simulink model "PassVeh3DOF"  (R2020a)
settings: Solver=ode4  StartTime=0.0  StopTime=10  FixedStep=.001  RelTol=3e-3
model workspace (MAT data in the model file):
  A_mu = 10
  B_reff = 8.386
  CONVERTER_DATA = [0 0.1 0.2 0.3 0.4 0.5 0.6 0.7 0.8 0.81 0.82 0.83 ... (63 elements, 21x3)]
  Cps = 2
  Cz = 7766.25
  DOWN_TABLE = [0 0 0 0 0 0 5 5 7.5 7.5 15 15 ... (30 elements, 6x5)]
  DOWN_TH_BP = [0 5 40 50 90 100]
  D_reff = 0.25826
  EMAP = [-40 215 245 264 264 267 267 267 267 267 -44 117 ... (110 elements, 10x11)]
  F0z = [6086.4 4324.8]
  F_reff = 0.07394
  F_zmax = 10000
  F_zmin = 100
  F_zo = 4000
  Kz = 48000
  MF : object (value not decoded)
  NCyl = 6
  NE_VEC = [800 1200 1600 2000 2400 2800 3200 3600 4000 4400 4800]
  Pstd = 101325
  Rair = 287
  SUS : object (value not decoded)
  TH_VEC = [0; 20; 30; 40; 50; 60; 70; 80; 90; 100]
  TWAITdn = 1.25
  TWAITup = 0.1
  Tin = [1 2 3 4 5 6 7 8 9 10 2 2 ... (20 elements, 10x2)]
  Tstd = 293.15
  UP_TABLE = [7.5 7.5 15 25 40 40 25 25 35 45 70 80 ... (30 elements, 6x5)]
  UP_TH_BP = [0 25 35 50 90 100]
  VEH : object (value not decoded)
  V_o = 16.7
  V_xlow = 1
  Vd = 0.00346
  WH : object (value not decoded)
  a = 1.4
  alpha_max = 1.5
  alpha_min = -1.5
  b = 1.8
  c_zo = 209651
  epsilon = 0.1
  f_air = [0 0 0 0 0 0 0 0 0 0 0 0 ... (256 elements, 16x16)]
  f_co = [0 0 0 0 0 0 0 0 0 0 0 0 ... (256 elements, 16x16)]
  f_co2 = [0 0 0 0 0 0 0 0 0 0 0 0 ... (256 elements, 16x16)]
  f_eff = [352.135682859 352.135682859 320.724378192 303.655312657 295.930136708 291.240087194 291.240271258 291.240312459 291.240275452 291.240198499 291.240100781 291.240018769 ... (256 elements, 16x16)]
  f_fuel = [0 0 0 0 0 0 0 0 0 0 0 0 ... (256 elements, 16x16)]
  f_hc = [0 0 0 0 0 0 0 0 0 0 0 0 ... (256 elements, 16x16)]
  f_nox = [0 0 0 0 0 0 0 0 0 0 0 0 ... (256 elements, 16x16)]
  f_pm = [0 0 0 0 0 0 0 0 0 0 0 0 ... (256 elements, 16x16)]
  f_susp_axl_bp = [1 2]
  f_susp_dz_bp = [-4 -0.14 -0.13 -0.12 -0.11 -0.1 -0.09 -0.08 -0.07 -0.06 -0.05 -0.04 ... (31 elements, 1x31)]
  f_susp_dzdot_bp = [-4 -0.14 -0.13 -0.12 -0.11 -0.1 -0.09 -0.08 -0.07 -0.06 -0.05 -0.04 ... (31 elements, 1x31)]
  f_susp_fmz = [-213379.591456 -28099.591456 -27619.591456 -27139.591456 -26659.591456 -26179.591456 -25699.591456 -25219.591456 -24739.591456 -24259.591456 -23779.591456 -23299.591456 ... (468968 elements, 31x31x61x2x4)]
  f_susp_geom = [-0.832564012244 0.043269987756 0.045538987756 0.047807987756 0.050076987756 0.052345987756 0.054614987756 0.056883987756 0.059152987756 0.061421987756 0.063690987756 0.065959987756 ... (11346 elements, 31x61x2x3)]
  f_susp_strgdelta_bp = [-0.523598775598 -0.506145483078 -0.488692190558 -0.471238898038 -0.453785605519 -0.436332312999 -0.418879020479 -0.401425727959 -0.383972435439 -0.366519142919 -0.349065850399 -0.331612557879 ... (61 elements, 1x61)]
  f_tbrake = [0 76.8593923996 105.140482948 131.533638111 157.926793274 176.658631717 176.65727296 176.656856686 176.656879077 176.657093756 176.657404516 176.65772406 ... (256 elements, 16x16)]
  f_tbrake_n_bpt = [0 649.519052838 912.419621844 1175.32019085 1438.22075986 1701.12132886 1964.02189787 2226.92246687 2489.82303588 2752.72360489 3015.62417389 3278.5247429 ... (16 elements, 1x16)]
  f_tbrake_t_bpt = [0 34.6410161514 61.0341713143 87.4273264773 113.82048164 140.213636803 166.606791966 192.999947129 219.393102292 245.786257455 272.179412618 298.572567781 ... (16 elements, 1x16)]
  f_texh = [766.752464599 766.752464599 786.17542386 801.679939032 884.591982581 910.574397722 910.571871054 910.570774534 910.570601632 910.570821151 910.571247242 910.571639815 ... (256 elements, 16x16)]
  f_twc_eff_co = [0.17 0.25 0.45 0.99 0.99 0.99 0.99]
  f_twc_eff_hc = [0.21 0.375 0.75 0.98 0.98 0.98 0.98]
  f_twc_eff_lam = [0.909090909 0.944055944 0.979020979 1 1.013986014 1.048951049 1.083916084]
  f_twc_eff_nox = [0.98 0.98 0.98 0.97 0.05 0.02 0]
  h = 0.5
  k_z = 50
  kappa_max = 1.5
  kappa_min = -1.5
  lam_Cx = 1
  lam_Cy = 1
  lam_Cz = 1
  lam_Ex = 1
  lam_Ey = 1
  lam_F_zo = 1
  lam_Hx = 1
  lam_Hy = 1
  lam_Kxkappa = 1
  lam_Kyalpha = 1
  lam_Kygamma = 1
  lam_Kzgamma = 1
  lam_Mr = 1
  lam_Mx = 1
  lam_My = 1
  lam_S = 1
  lam_VMx = 1
  lam_Vx = 1
  lam_Vy = 1
  lam_Vykappa = 1
  lam_muV = 0
  lam_mux = 1
  lam_muy = 1
  lam_t = 1
  lam_xalpha = 1
  lam_ykappa = 1
  numWheel = 4
  p_Cx1 = 1.579
  p_Cy1 = 1.3332
  p_Dx1 = 1.0422
  p_Dx2 = -0.08285
  p_Dx3 = 0
  p_Dy1 = 0.8784
  p_Dy2 = -0.06445
  p_Dy3 = 0
  p_Ex1 = 0.11185
  p_Ex2 = 0.3127
  p_Ex3 = 0
  p_Ex4 = 0.001603
  p_Ey1 = -0.8227
  p_Ey2 = -0.6062
  p_Ey3 = 0.09825
  p_Ey4 = -6.546
  p_Ey5 = 0
  p_Fz1 = 0.7098
  p_Hx1 = 0.00021585
  p_Hx2 = 0.0011538
  p_Hy1 = -0.0018043
  p_Hy2 = 0.003518
  p_Kx1 = 21.69
  p_Kx2 = 13.774
  p_Kx3 = -0.4119
  p_Ky1 = -15.314
  p_Ky2 = 1.7044
  p_Ky3 = 0.36986
  p_Ky4 = 1.9896
  p_Ky5 = 0
  p_Ky6 = -0.9004
  p_Ky7 = -0.2328
  p_Vx1 = 1.5973e-05
  p_Vx2 = 0.0001043
  p_Vy1 = -0.006642
  p_Vy2 = 0.03597
  p_Vy3 = -0.1621
  p_Vy4 = -0.4908
  p_pmx1 = 0
  p_px1 = -0.3489
  p_px2 = 0.382
  p_px3 = -0.09634
  p_px4 = 0.06447
  p_py1 = -0.6249
  p_py2 = -0.06535
  p_py3 = -0.1668
  p_py4 = 0.2834
  p_py5 = 0
  path : object (value not decoded)
  pio = 220000
  q_Fcx = 0
  q_Fz2 = 15.4
  q_Fzy = 0
  q_reo = 0.9974
  q_sx1 = -0.007764
  q_sx10 = 0.2824
  q_sx11 = 5.349
  q_sx12 = 0
  q_sx13 = 0
  q_sx14 = 0
  q_sx2 = 1.1915
  q_sx3 = 0.013948
  q_sx4 = 4.912
  q_sx5 = 1.02
  q_sx6 = 22.83
  q_sx7 = 0.7104
  q_sx8 = -0.023393
  q_sx9 = 0.6581
  q_sy1 = 0.00702
  q_sy2 = 0
  q_sy3 = 0.001515
  q_sy4 = 8.514e-05
  q_sy5 = 0
  q_sy6 = 0
  q_sy7 = 0.9008
  q_sy8 = -0.4089
  q_v1 = 0.0007742
  q_v2 = 0.04667
  r_Bx1 = 12.531
  r_Bx2 = 9.532
  r_Bx3 = 0
  r_By1 = 10.615
  r_By2 = 7.705
  r_By3 = 3.433e-06
  r_By4 = 0
  r_Cx1 = 1.019
  r_Cy1 = 1.0585
  r_Ex1 = -0.4487
  r_Ex2 = -0.4726
  r_Ey1 = 0.3132
  r_Ey2 = 7.63e-06
  r_Hx1 = 0.0002374
  r_Hy1 = 0.011646
  r_Hy2 = 7.63e-06
  r_Vy1 = 0.05654
  r_Vy2 = 7.63e-06
  r_Vy3 = 0
  r_Vy4 = 99.9
  r_Vy5 = 2
  r_Vy6 = 15.814
  r_o = 0.3135
  reqTmaxT = [nan 0.285774810084 0.647179872268 nan nan nan nan nan nan nan nan nan ... (168 elements, 21x8)]
  vehSpd = [0 2.77777777778 5.55555555556 8.33333333333 11.1111111111 13.8888888889 16.6666666667 19.4444444444 22.2222222222 25 27.7777777778 30.5555555556 ... (21 elements, 1x21)]
  vehWidth = 2
  w = 1
libraries: autolibutils x4, autolibshared x2, simulink x1, vehdynlibsteering x1
(part 4 of 4)

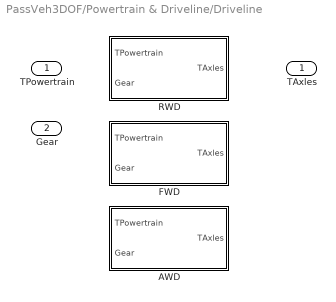
== system PassVeh3DOF/Powertrain & Driveline/Driveline ==
  TPowertrain : Inport
  Gear : Inport  Port=2
  AWD : Subsystem  VariantControl=2
  FWD : Subsystem  VariantControl=1
  RWD : Subsystem  VariantControl=0
  TAxles : Outport  VectorParamsAs1DForOutWhenUnconnected=off

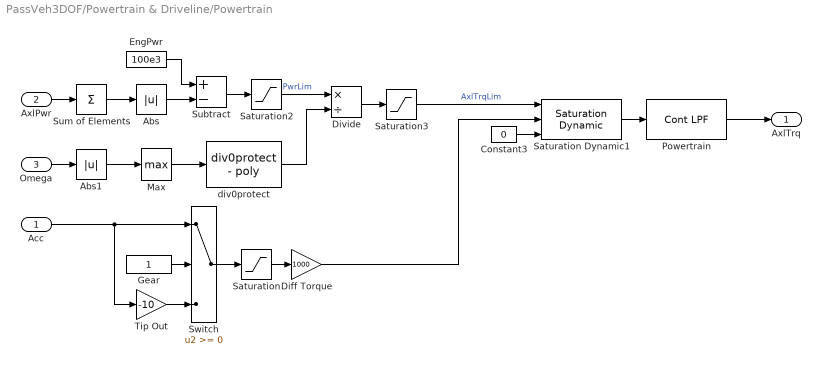
== system PassVeh3DOF/Powertrain & Driveline/Powertrain ==
  Acc : Inport
  AxlPwr : Inport  Port=2
  Omega : Inport  Port=3
  Abs : Abs  ZeroCross=off
  Abs1 : Abs  ZeroCross=off
  Constant3 : Constant  Value=0
  Diff Torque : Gain  Gain=1000
  Divide : Product  Inputs=*/
  EngPwr : Constant  Value=100e3
  Gear : Constant  SampleTime=-1
  Max : MinMax  Function=max  ZeroCross=off
  Powertrain : autolibutils/Cont LPF  wc=4*pi*2  aMode=2
      settings: SourceProductBaseCode=PW,MT,VE,VP
  Saturation : Saturate  UpperLimit=inf  LowerLimit=0  ZeroCross=off
  Saturation Dynamic1 : simulink/Discontinuities/Saturation Dynamic  OutMin=[]  OutMax=[]  OutDataTypeStr=Inherit: Same as second input  OutDataType=fixdt(1, 16)  OutScaling=2^-10  DoSatur=off
  Saturation2 : Saturate  UpperLimit=inf  LowerLimit=100  ZeroCross=off
  Saturation3 : Saturate  UpperLimit=1000  LowerLimit=0  ZeroCross=off
  Subtract : Sum  Inputs=+-
  Sum of Elements : Sum  Inputs=+
  Switch : Switch  ZeroCross=off
  Tip Out : Gain  Gain=-10
  div0protect : autolibutils/div0protect - poly  thresh=1  aMode=2
      settings: SourceProductBaseCode=PW,MT,VE,VP
  AxlTrq : Outport  VectorParamsAs1DForOutWhenUnconnected=off
  wires:
  Powertrain/1 -> AxlTrq/1
  Switch/1 -> Saturation/1
  Acc/1 -> Tip Out/1, Switch/1
  Saturation/1 -> Diff Torque/1
  Diff Torque/1 -> Saturation Dynamic1/2
  Gear/1 -> Switch/2
  Saturation Dynamic1/1 -> Powertrain/1
  Tip Out/1 -> Switch/3
  Constant3/1 -> Saturation Dynamic1/3
  Sum of Elements/1 -> Abs/1
  Abs/1 -> Subtract/2
  Divide/1 -> Saturation3/1
  div0protect/1 -> Divide/2
  Omega/1 -> Abs1/1
  Subtract/1 -> Saturation2/1
  Saturation2/1 -> Divide/1  "PwrLim"
  EngPwr/1 -> Subtract/1
  AxlPwr/1 -> Sum of Elements/1
  Saturation3/1 -> Saturation Dynamic1/1  "AxlTrqLim"
  Max/1 -> div0protect/1
  Abs1/1 -> Max/1

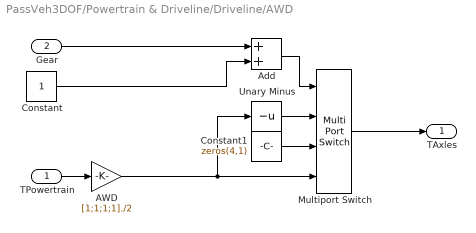
== system PassVeh3DOF/Powertrain & Driveline/Driveline/AWD ==
  TPowertrain : Inport
  Gear : Inport  Port=2
  AWD : Gain  Gain=[1;1;1;1]./2
  Add : Sum
  Constant : Constant
  Constant1 : Constant  Value=zeros(4,1)
  Multiport Switch : MultiPortSwitch  DataPortOrder=Zero-based contiguous  zeroidx=on
  Unary Minus : UnaryMinus
  TAxles : Outport  VectorParamsAs1DForOutWhenUnconnected=off
  wires:
  TPowertrain/1 -> AWD/1
  Multiport Switch/1 -> TAxles/1
  Add/1 -> Multiport Switch/1
  Constant1/1 -> Multiport Switch/3
  AWD/1 -> Unary Minus/1, Multiport Switch/4
  Constant/1 -> Add/2
  Gear/1 -> Add/1
  Unary Minus/1 -> Multiport Switch/2

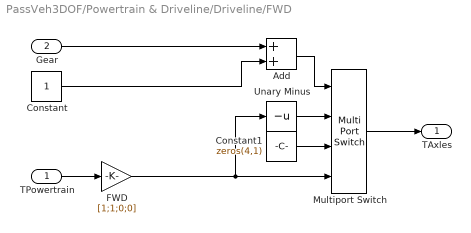
== system PassVeh3DOF/Powertrain & Driveline/Driveline/FWD ==
  TPowertrain : Inport
  Gear : Inport  Port=2
  Add : Sum
  Constant : Constant
  Constant1 : Constant  Value=zeros(4,1)
  FWD : Gain  Gain=[1;1;0;0]
  Multiport Switch : MultiPortSwitch  DataPortOrder=Zero-based contiguous  zeroidx=on
  Unary Minus : UnaryMinus
  TAxles : Outport  VectorParamsAs1DForOutWhenUnconnected=off
  wires:
  TPowertrain/1 -> FWD/1
  Multiport Switch/1 -> TAxles/1
  Add/1 -> Multiport Switch/1
  Constant1/1 -> Multiport Switch/3
  FWD/1 -> Unary Minus/1, Multiport Switch/4
  Constant/1 -> Add/2
  Gear/1 -> Add/1
  Unary Minus/1 -> Multiport Switch/2

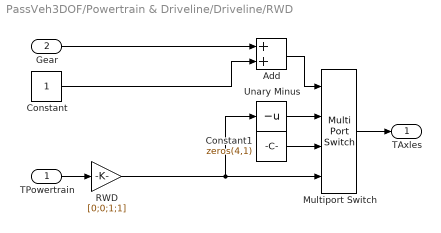
== system PassVeh3DOF/Powertrain & Driveline/Driveline/RWD ==
  TPowertrain : Inport
  Gear : Inport  Port=2
  Add : Sum
  Constant : Constant
  Constant1 : Constant  Value=zeros(4,1)
  Multiport Switch : MultiPortSwitch  DataPortOrder=Zero-based contiguous  zeroidx=on
  RWD : Gain  Gain=[0;0;1;1]
  Unary Minus : UnaryMinus
  TAxles : Outport  VectorParamsAs1DForOutWhenUnconnected=off
  wires:
  RWD/1 -> Unary Minus/1, Multiport Switch/4
  TPowertrain/1 -> RWD/1
  Unary Minus/1 -> Multiport Switch/2
  Multiport Switch/1 -> TAxles/1
  Gear/1 -> Add/1
  Constant/1 -> Add/2
  Add/1 -> Multiport Switch/1
  Constant1/1 -> Multiport Switch/3
